simulink model "prop_tilt_gyro_model_1"  (R2020b)
settings: Solver=VariableStepAuto  StartTime=0.0  StopTime=T_prop  RelTol=1e-3
values from neighbouring files (symbols this model uses):
  I_mat = I_diag    [Propellers_tilt.m]    (also in six.m = Inertia; tilt_verification.m = 0)
  psI_0 = 0    [Propellers_tilt.m]    (also in tilt_verification.m)
  w_p_0 = 90*pi/(180*T_prop)    (= 1.57079632679)    [Propellers_tilt.m]    (also in tilt_verification.m)
  w_p_dot = 0    [Propellers_tilt.m]    (also in tilt_verification.m)
  w_s_0 = 3500*2*pi/2    (= 10995.5742876)    [Propellers_tilt.m]    (also in tilt_verification.m)
  w_s_dot = 0    [Propellers_tilt.m]    (also in tilt_verification.m)
libraries: sharedutil x1
settings Model: Creator=Jonathan van Zyl  LastModifiedBy=Jonathan van Zyl

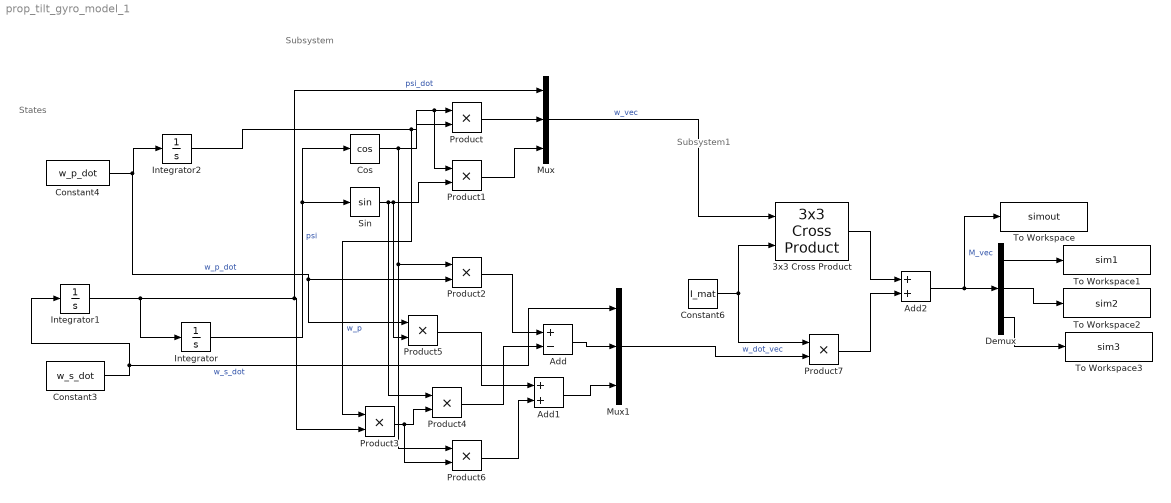
== system prop_tilt_gyro_model_1 ==
  note: Subsystem1
  note: Subsystem
  note: States
  3x3 Cross Product : sharedutil/3x3 Cross Product  aMode=aMode
      settings: SourceProductBaseCode=AE,PW,MT,UV,VE,VP
  Add : Sum  Inputs=+-
  Add1 : Sum
  Add2 : Sum
  Constant3 : Constant  Value=w_s_dot
  Constant4 : Constant  Value=w_p_dot
  Constant6 : Constant  Value=I_mat
  Cos : Trigonometry  Operator=cos
  Demux : Demux  Outputs=3
  Integrator : Integrator  InitialCondition=psI_0
  Integrator1 : Integrator  InitialCondition=w_s_0
  Integrator2 : Integrator  InitialCondition=w_p_0
  Mux : Mux  Inputs=3
  Mux1 : Mux  Inputs=3
  Product{,1..7} (8 alike) : Product
  Sin : Trigonometry
  To Workspace : ToWorkspace  VariableName=simout  SaveFormat=Timeseries  SampleTime=-1
  To Workspace1 : ToWorkspace  VariableName=sim1  SampleTime=-1
  To Workspace2 : ToWorkspace  VariableName=sim2  SaveFormat=Timeseries  SampleTime=-1
  To Workspace3 : ToWorkspace  VariableName=sim3  SaveFormat=Timeseries  SampleTime=-1
  wires:
  Demux/1 -> To Workspace1/1
  Demux/2 -> To Workspace2/1
  Demux/3 -> To Workspace3/1
  Constant3/1 -> Integrator1/1, Mux1/1  "w_s_dot"
  Constant4/1 -> Integrator2/1, Product5/1, Product2/2  "w_p_dot"
  Integrator/1 -> Cos/1, Sin/1  "psi"
  Integrator1/1 -> Mux/1, Product3/2, Integrator/1  "psi_dot"
  Integrator2/1 -> Product1/1, Product/1, Product3/1  "w_p"
  Mux1/1 -> Product7/2  "w_dot_vec"
  Product1/1 -> Mux/3
  Product4/1 -> Add/2
  Product5/1 -> Add1/1
  Mux/1 -> 3x3 Cross Product/1  "w_vec"
  Product/1 -> Mux/2
  Add1/1 -> Mux1/3
  Product6/1 -> Add1/2
  Sin/1 -> Product4/1, Product5/2, Product1/2
  Cos/1 -> Product6/1, Product2/1, Product/2
  Product2/1 -> Add/1
  Product3/1 -> Product6/2, Product4/2
  Add/1 -> Mux1/2
  Add2/1 -> Demux/1, To Workspace/1  "M_vec"
  3x3 Cross Product/1 -> Add2/1
  Constant6/1 -> Product7/1, 3x3 Cross Product/2
  Product7/1 -> Add2/2
